simulink model "regulatorP"  (R2021b)
settings: Solver=VariableStepAuto  StartTime=0.0  StopTime=500  RelTol=1e-3
model workspace (MAT data in the model file):
  zmienna1 = [2 4 10 1]
settings Model: SnapshotBufferSize=50  Creator=mateusznowak  LastModifiedBy=mateusznowak

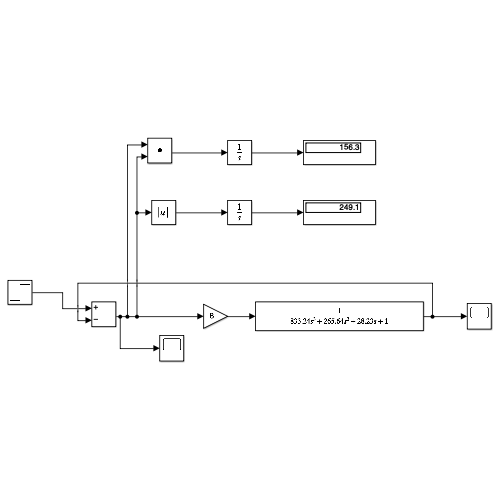
[thumbnail: Simulink's stored preview of the top-level diagram]
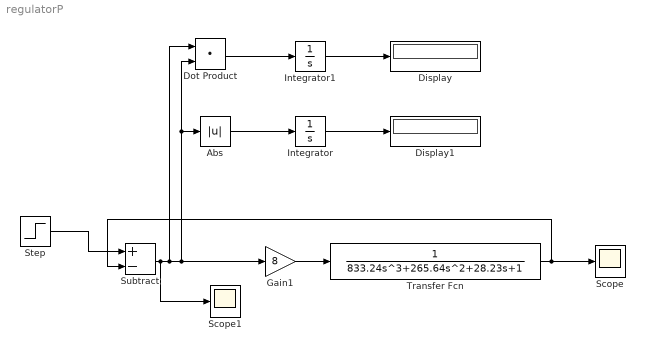
== system regulatorP ==
  Abs : Abs
  Display : Display
  Display1 : Display
  Dot Product : DotProduct  InputSameDT=on  OutDataTypeStr=Inherit: Inherit via internal rule
  Gain1 : Gain  Gain=8
  Integrator : Integrator
  Integrator1 : Integrator
  Scope : Scope
  Scope1 : Scope
  Step : Step  SampleTime=0
  Subtract : Sum  Inputs=+-
  Transfer Fcn : TransferFcn  Denominator=[833.24 265.64 28.23 1]
  wires:
  Step/1 -> Subtract/1
  Subtract/1 -> Scope1/1, Dot Product/1, Gain1/1, Dot Product/2, Abs/1
  Gain1/1 -> Transfer Fcn/1
  Transfer Fcn/1 -> Scope/1, Subtract/2
  Abs/1 -> Integrator/1
  Integrator/1 -> Display1/1
  Dot Product/1 -> Integrator1/1
  Integrator1/1 -> Display/1
